simulink model "afe_abc_inv_psm_2mods"  (R2025b)
settings: Solver=ode1  StartTime=0.0  StopTime=simlength  FixedStep=tc  MaxStep=tc
values from neighbouring files (symbols this model uses):
  Adrso = eye(2) + Arso*ts_afe    [init_model.m]
  afe_pwm_phase_shift_mod1 = 0    [init_model.m]
  afe_pwm_phase_shift_mod2 = 0    [init_model.m]
  Aresd = eye(2) + Ares*ts_afe    [init_model.m]
  Bresd = Bres*ts_afe    [init_model.m]
  Cresd = Cres    [init_model.m]
  Crso = [1 0]    [init_model.m]
  CTRPIFF_CLIP_RELEASE = 0.001    [init_model.m]
  dead_time_AFE = 3e-6    (= 3e-06)    [init_model.m]
  dead_time_INV = 3e-6    (= 3e-06)    [init_model.m]
  deepNEGeta = 0.5    [init_model.m]
  deepNEGxi = 0    [init_model.m]
  deepPOSxi = 0.5    [init_model.m]
  emf_fb_p = 0.2    [init_model.m]
  emf_fb_p_ccaller_1 = emf_fb_p    (= 0.2)    [init_model.m]
  emf_fb_p_ccaller_2 = emf_fb_p    (= 0.2)    [init_model.m]
  emf_p = emf_fb_p*4/10    (= 0.08)    [init_model.m]
  emf_p_ccaller_1 = emf_fb_p_ccaller_1*4/10    (= 0.08)    [init_model.m]
  emf_p_ccaller_2 = emf_fb_p_ccaller_2*4/10    (= 0.08)    [init_model.m]
  fPWM_AFE = 4e3    (= 4000)    [init_model.m]
  fPWM_INV = fPWM_AFE    (= 4000)    [init_model.m]
  g0_161Hz = fcut_161Hz_flt * ts_afe * 2*pi    (= 0.126449104307)    [init_model.m]
  g0_1Hz = fcut_1Hz_flt * ts_afe * 2*pi    (= 0.000785398163397)    [init_model.m]
  g0_500Hz = fcut_500Hz_flt * ts_afe * 2*pi    (= 0.392699081699)    [init_model.m]
  g1_161Hz = 1 - g0_161Hz    (= 0.873550895693)    [init_model.m]
  g1_1Hz = 1 - g0_1Hz    (= 0.999214601837)    [init_model.m]
  g1_500Hz = 1 - g0_500Hz    (= 0.607300918301)    [init_model.m]
  i_grid_neg_eta_lim = 0.5    [init_model.m]
  i_grid_neg_eta_red_lim = 0.1    [init_model.m]
  i_grid_neg_xi_lim = 0.5    [init_model.m]
  i_grid_neg_xi_red_lim = 0.1    [init_model.m]
  i_grid_pos_eta_lim = 1    [init_model.m]
  i_grid_pos_eta_red_lim = 0.1    [init_model.m]
  id_lim = 0.35    [init_model.m]
  ieta_neg_ref_lim = 0.5    [init_model.m]
  ieta_pos_ref_lim = 1.0    (= 1)    [init_model.m]
  Igrid_phase_normalization_factor = 250e3/Vphase2/3/0.9*sqrt(2)    [init_model.m]
  inv_pwm_phase_shift_mod1 = 0    [init_model.m]
  iq_lim = 1.4    [init_model.m]
  ixi_pos_ref_lim = 1.6    [init_model.m]
  k_frt_ref = 2    [init_model.m]
  kg = Kobs(1)    [init_model.m]
  ki_afe = 45    [init_model.m]
  ki_align = 0.1    [init_model.m]
  ki_i = 18    [init_model.m]
  ki_rc_neg_grid = ki_rc_grid    (= 35)    [init_model.m]
  ki_rc_pos_grid = ki_rc_grid    (= 35)    [init_model.m]
  ki_vs = 35    [init_model.m]
  ki_w = 18    [init_model.m]
  kp_afe = 0.6    [init_model.m]
  kp_align = 0.6    [init_model.m]
  kp_i = 0.25    [init_model.m]
  kp_rc_neg_grid = kp_rc_grid    (= 0.35)    [init_model.m]
  kp_rc_pos_grid = kp_rc_grid    (= 0.35)    [init_model.m]
  kp_vs = 0.85    [init_model.m]
  kp_w = 2.5    [init_model.m]
  kw = Kobs(2)    [init_model.m]
  l1 = Kd(2)    [init_model.m]
  l2 = Kd(1)    [init_model.m]
  Ldrso = acker(Adrso',Crso',polesdrso)'    [init_model.m]
  lim_down_align = -0.2    [init_model.m]
  lim_up_align = 0.2    [init_model.m]
  mavarage_filter_frequency_base_order = 2    [init_model.m]
  motorc_m_scale = 2/3*Vdc_bez/ubez    [init_model.m]
  n1 = rms_perios/f_grid/ts_afe    [init_model.m]
  n10 = rms_perios/f_grid/ts_afe    [init_model.m]
  number_of_modules = 2    [init_model.m]
  omega_m_sim = omega_m_bez    [init_model.m]
  pll_i1 = 80    [init_model.m]
  pll_i1_ddsrt = pll_i1/2    (= 40)    [init_model.m]
  pll_p = 1    [init_model.m]
  pll_p_ddsrt = pll_p/2    (= 0.5)    [init_model.m]
  pll_p_frt = 0.2    [init_model.m]
  settle_time = 0.15    [init_model.m]
  simlength = 2    [init_model.m]
  start_time_LVRT = 2.0    (= 2)    [init_model.m]
  tc = ts_afe/200    (= 6.25e-07)    [init_model.m]
  time_aux_power_supply_fault = 1e3    (= 1000)    [init_model.m]
  time_gain_afe_module_1 = 1.0    (= 1)    [init_model.m]
  time_gain_afe_module_2 = 1.0    (= 1)    [init_model.m]
  time_gain_inv_module_1 = 1.0    (= 1)    [init_model.m]
  time_gain_inv_module_2 = 1.0    (= 1)    [init_model.m]
  time_phase_fault = 1e3    (= 1000)    [init_model.m]
  time_start_motor_control = 0.035    [init_model.m]
  transmission_delay = 125e-6*2    (= 0.00025)    [init_model.m]
  ts_afe = 1/fPWM_AFE/2    (= 0.000125)    [init_model.m]
  ts_inv = 1/fPWM_INV/2    (= 0.000125)    [init_model.m]
  Vdc_norm_ref = Vdc_ref/Vdc_nom    [init_model.m]
  Vdc_ref = 1070    [init_model.m]
  Vgrid_phase_normalization_factor = Vphase2*sqrt(2)    [init_model.m]
  w_grid = 2*pi*f_grid    [init_model.m]
undefined symbols (not defined in the file or in its folder): Amplitude_U, Amplitude_V, Amplitude_W, end_time_LVRT, ibez, La, Lb, Ld_norm, Lq_norm, Ls_norm, magnitude, omega_bez, omega_grid_emulator_nom, omega_grid_nom, omega_m_bez, Phase_shift, psi_bez, psi_m, psi_m_norm, rpm_base, rpm_bez, Rs, Rs_norm, t_ramp, tau_bez, torque_base, ubez, ugrid_factor, V_phase_normalization_factor, Vdc_bez, Vemu_ref_norm, vn_eta_pu, vn_xi_pu, vp_xi_pu
libraries: fl_lib x215, nesl_utility x107, simulink x22, cstblocks x20, threephase_inductor_lib x4, single_phase_transformer_lib x3, flexshaft_lib x1, psm x1
(part 9 of 19)

== system afe_abc_inv_psm_2mods/afe_abc_inv_psm_mod2/AFE_control/afe_control/FRT-VDE4110/FRT-Detection ==
  red_dyn_enabled : Inport
  Abs : Abs  SaturateOnIntegerOverflow=off
  Abs1 : Abs  SaturateOnIntegerOverflow=off
  LVRT_detector : MATLAB Function  TreatAsAtomicUnit=on
  Step1 : Step  Time=0.025  Before=1  After=0
  Step3 : Step  Time=settle_time
  dvxi_n/dt : Subsystem
  dvxi_p/dt : Subsystem
  frt_detection_inputs mod2 : Scope  NumInputPorts=6
      settings: ActiveDisplayYMinimum=-0.12991  ActiveDisplayYMaximum=1.13961  DataLoggingVariableName=ScopeData2
  frt_exceeded : Outport
  frt_state : Outport  Port=2
  red_dyn_active : Outport  Port=3
  frt_active : Outport  Port=4
  pwr_lim_enable : Outport  Port=5
  wires:
  Abs1/1 -> LVRT_detector/5(vxi_n_dot), frt_detection_inputs mod2/5  "vxi_neg_dot"
  Abs/1 -> LVRT_detector/4(vxi_p_dot), frt_detection_inputs mod2/4  "vxi_pos_dot"
  LVRT_detector/3(frt_active) -> frt_active/1
  LVRT_detector/4(frt_state) -> frt_state/1
  LVRT_detector/5(red_dyn_active) -> red_dyn_active/1
  LVRT_detector/2(frt_exceeded) -> frt_exceeded/1  "lvrt_exceeded"
  red_dyn_enabled/1 -> LVRT_detector/7(red_dyn_enabled)
  Step1/1 -> LVRT_detector/8(reset)
  dvxi_n/dt/1(xdot_hat) -> Abs1/1
  LVRT_detector/1(pwr_lim_enable) -> pwr_lim_enable/1  "pwr_lim_enable"
  dvxi_p/dt/1(xdot_hat) -> Abs/1
  Step3/1 -> LVRT_detector/6(enable), frt_detection_inputs mod2/6  "enable"
  [v_grid_neg_eta_avg_mod2] -> frt_detection_inputs mod2/3, LVRT_detector/3(veta_n)  "v_grid_neg_eta_avg"
  [v_grid_pos_xi_avg_mod2] -> dvxi_p/dt/1(x), frt_detection_inputs mod2/1, LVRT_detector/1(vxi_p)  "v_grid_pos_xi_avg"
  [v_grid_neg_xi_avg_mod2] -> dvxi_n/dt/1(x), frt_detection_inputs mod2/2, LVRT_detector/2(vxi_n)  "v_grid_neg_xi_avg"

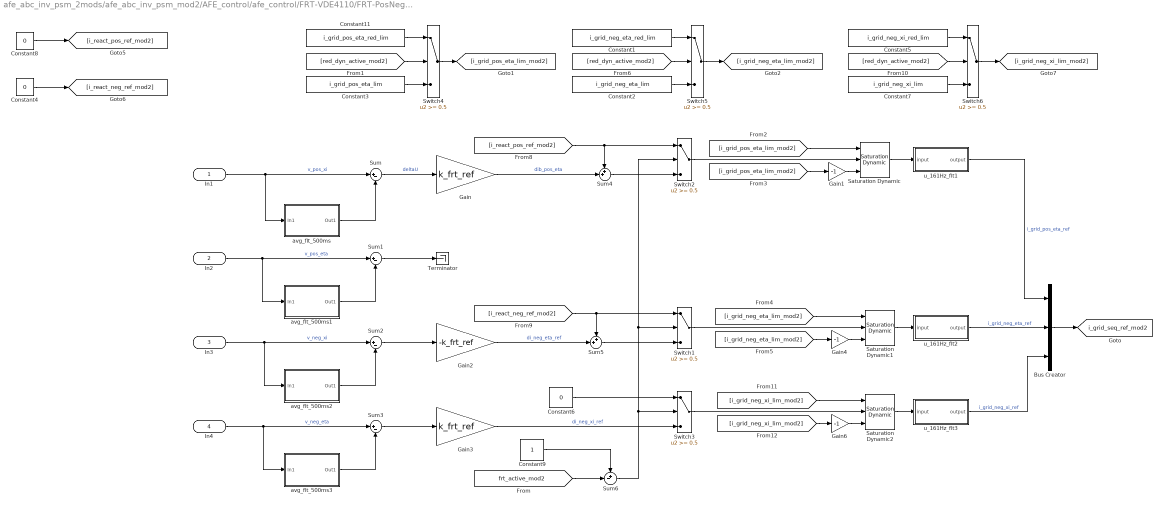
== system afe_abc_inv_psm_2mods/afe_abc_inv_psm_mod2/AFE_control/afe_control/FRT-VDE4110/FRT-PosNegReactiveCurrentReferences ==
  In1 : Inport
  In2 : Inport  Port=2
  In3 : Inport  Port=3
  In4 : Inport  Port=4
  Bus Creator : BusCreator  Inputs=3
  Constant1 : Constant  Value=i_grid_neg_eta_red_lim
  Constant11 : Constant  Value=i_grid_pos_eta_red_lim
  Constant2 : Constant  Value=i_grid_neg_eta_lim
  Constant3 : Constant  Value=i_grid_pos_eta_lim
  Constant4 : Constant  Value=0
  Constant5 : Constant  Value=i_grid_neg_xi_red_lim
  Constant6 : Constant  Value=0
  Constant7 : Constant  Value=i_grid_neg_xi_lim
  Constant8 : Constant  Value=0
  Constant9 : Constant
  Gain : Gain  Gain=k_frt_ref
  Gain1 : Gain  Gain=-1
  Gain2 : Gain  Gain=-k_frt_ref
  Gain3 : Gain  Gain=k_frt_ref
  Gain4 : Gain  Gain=-1
  Gain6 : Gain  Gain=-1
  Saturation Dynamic : simulink/Discontinuities/Saturation Dynamic  OutMin=[]  OutMax=[]  OutDataTypeStr=Inherit: Same as second input  OutDataType=fixdt(1, 16)  OutScaling=2^-10  DoSatur=off
  Saturation Dynamic1 : simulink/Discontinuities/Saturation Dynamic  OutMin=[]  OutMax=[]  OutDataTypeStr=Inherit: Same as second input  OutDataType=fixdt(1, 16)  OutScaling=2^-10  DoSatur=off
  Saturation Dynamic2 : simulink/Discontinuities/Saturation Dynamic  OutMin=[]  OutMax=[]  OutDataTypeStr=Inherit: Same as second input  OutDataType=fixdt(1, 16)  OutScaling=2^-10  DoSatur=off
  Sum{,1..3} (4 alike) : Sum  Inputs=|+-
  Sum4 : Sum  Inputs=++|
  Sum5 : Sum  Inputs=++|
  Sum6 : Sum  Inputs=+-|
  Switch{1..6} (6 alike) : Switch  Threshold=0.5  SaturateOnIntegerOverflow=off  InputSameDT=off
  Terminator : Terminator
  avg_flt_500ms : Subsystem
  avg_flt_500ms1 : Subsystem
  avg_flt_500ms2 : Subsystem
  avg_flt_500ms3 : Subsystem
  u_161Hz_flt1 : Subsystem
  u_161Hz_flt2 : Subsystem
  u_161Hz_flt3 : Subsystem
  tag scope: i_grid_seq_ref_mod2=global
  wires:
  Constant9/1 -> Sum6/1
  [frt_active_mod2] -> Sum6/2
  u_161Hz_flt1/1(output) -> Bus Creator/1  "i_grid_pos_eta_ref"
  u_161Hz_flt3/1(output) -> Bus Creator/3  "i_grid_neg_xi_ref"
  u_161Hz_flt2/1(output) -> Bus Creator/2  "i_grid_neg_eta_ref"
  Gain6/1 -> Saturation Dynamic2/3
  [red_dyn_active_mod2] -> Switch6/2
  Constant5/1 -> Switch6/1
  Switch6/1 -> [i_grid_neg_xi_lim_mod2]
  Constant7/1 -> Switch6/3
  Constant8/1 -> [i_react_pos_ref_mod2]
  Constant4/1 -> [i_react_neg_ref_mod2]
  Switch5/1 -> [i_grid_neg_eta_lim_mod2]
  Constant1/1 -> Switch5/1
  Constant2/1 -> Switch5/3
  [red_dyn_active_mod2] -> Switch5/2
  Saturation Dynamic1/1 -> u_161Hz_flt2/1(input)
  Switch1/1 -> Saturation Dynamic1/2
  [i_grid_neg_eta_lim_mod2] -> Saturation Dynamic1/1
  [i_grid_neg_eta_lim_mod2] -> Gain4/1
  Gain4/1 -> Saturation Dynamic1/3
  [i_grid_neg_xi_lim_mod2] -> Gain6/1
  [i_grid_neg_xi_lim_mod2] -> Saturation Dynamic2/1
  Switch3/1 -> Saturation Dynamic2/2
  Saturation Dynamic2/1 -> u_161Hz_flt3/1(input)
  Gain1/1 -> Saturation Dynamic/3
  [i_grid_pos_eta_lim_mod2] -> Gain1/1
  [i_grid_pos_eta_lim_mod2] -> Saturation Dynamic/1
  Constant11/1 -> Switch4/1
  Constant3/1 -> Switch4/3
  [red_dyn_active_mod2] -> Switch4/2
  Switch4/1 -> [i_grid_pos_eta_lim_mod2]
  [i_react_neg_ref_mod2] -> Sum5/1, Switch1/1
  Sum5/1 -> Switch1/3
  Gain2/1 -> Sum5/2  "di_neg_eta_ref"
  Sum3/1 -> Gain3/1
  Sum6/1 -> Switch3/2, Switch2/2, Switch1/2
  Gain3/1 -> Switch3/3  "di_neg_xi_ref"
  Constant6/1 -> Switch3/1
  Saturation Dynamic/1 -> u_161Hz_flt1/1(input)
  Switch2/1 -> Saturation Dynamic/2
  Sum4/1 -> Switch2/3
  [i_react_pos_ref_mod2] -> Sum4/1, Switch2/1
  Gain/1 -> Sum4/2  "dib_pos_eta"
  Bus Creator/1 -> [i_grid_seq_ref_mod2]
  In4/1 -> Sum3/1, avg_flt_500ms3/1(In1)  "v_neg_eta"
  avg_flt_500ms2/1(Out1) -> Sum2/2
  In3/1 -> Sum2/1, avg_flt_500ms2/1(In1)  "v_neg_xi"
  Sum2/1 -> Gain2/1
  avg_flt_500ms3/1(Out1) -> Sum3/2
  In2/1 -> Sum1/1, avg_flt_500ms1/1(In1)  "v_pos_eta"
  avg_flt_500ms1/1(Out1) -> Sum1/2
  Sum1/1 -> Terminator/1
  Sum/1 -> Gain/1  "deltaU"
  avg_flt_500ms/1(Out1) -> Sum/2
  In1/1 -> Sum/1, avg_flt_500ms/1(In1)  "v_pos_xi"

== system afe_abc_inv_psm_2mods/afe_abc_inv_psm_mod2/AFE_control/afe_control/current_ctrl/Inner Loop Current Control ==
  In1 : Inport
  is_abc : Inport  Port=2
  -1<x<1 : Saturate  UpperLimit=1  LowerLimit=-1
  Add : Sum
  Bus Creator1 : BusCreator  Inputs=2
  "Current-Control, Phase a" : Subsystem
  "Current-Control, Phase b" : Subsystem
  "Current-Control, Phase c" : Subsystem
  Demux1 : Demux  Outputs=3
  MATLAB Function : MATLAB Function  TreatAsAtomicUnit=on
  Mux : Mux  Inputs=3
  Selector : Selector  InputPortWidth=3  IndexOptions=Index vector (dialog)  Indices=[1]  OutputSizes=1
  Selector1 : Selector  InputPortWidth=3  IndexOptions=Index vector (dialog)  Indices=[1]  OutputSizes=1
  Selector2 : Selector  InputPortWidth=3  IndexOptions=Index vector (dialog)  Indices=[2]  OutputSizes=1
  Selector3 : Selector  InputPortWidth=3  IndexOptions=Index vector (dialog)  Indices=[2]  OutputSizes=1
  Selector4 : Selector  InputPortWidth=3  IndexOptions=Index vector (dialog)  Indices=[3]  OutputSizes=1
  Selector5 : Selector  InputPortWidth=3  IndexOptions=Index vector (dialog)  Indices=[3]  OutputSizes=1
  To Workspace1 : ToWorkspace  VariableName=isa_ref_sim_mod2  SampleTime=-1
      settings: MaxDataPoints=Ns_afe
  To Workspace2 : ToWorkspace  VariableName=isa_sim_mod2  SampleTime=-1
      settings: MaxDataPoints=Ns_afe
  To Workspace3 : ToWorkspace  VariableName=isb_ref_sim_mod2  SampleTime=-1
      settings: MaxDataPoints=Ns_afe
  To Workspace4 : ToWorkspace  VariableName=isb_sim_mod2  SampleTime=-1
      settings: MaxDataPoints=Ns_afe
  To Workspace5 : ToWorkspace  VariableName=isc_ref_sim_mod2  SampleTime=-1
      settings: MaxDataPoints=Ns_afe
  To Workspace6 : ToWorkspace  VariableName=isc_sim_mod2  SampleTime=-1
      settings: MaxDataPoints=Ns_afe
  Unit Delay1 : UnitDelay  SampleTime=-1  HasFrameUpgradeWarning=on
  Unit Delay2 : UnitDelay  SampleTime=-1  HasFrameUpgradeWarning=on
  Unit Delay3 : UnitDelay  SampleTime=-1  HasFrameUpgradeWarning=on
  afe_ictrl_out/afe_ictrl_ff : Scope  NumInputPorts=2
      settings: ActiveDisplayYMinimum=-1.2844276731305864  ActiveDisplayYMaximum=1.2966894715372321  DataLoggingVariableName=ScopeData4
  isa_ref/isa : Scope  NumInputPorts=2
      settings: ActiveDisplayYMinimum=-1.06078125  ActiveDisplayYMaximum=1.00328125
  isb_ref/isb : Scope  NumInputPorts=2
      settings: ActiveDisplayYMinimum=-1.080322265625  ActiveDisplayYMaximum=1.007080078125  DataLoggingVariableName=ScopeData2
  isc_ref/isc : Scope  NumInputPorts=2
      settings: ActiveDisplayYMinimum=-1.005859375  ActiveDisplayYMaximum=1.0791015625  DataLoggingVariableName=ScopeData3
  uab : Outport  VectorParamsAs1DForOutWhenUnconnected=off
  wires:
  [isc_mod2] -> To Workspace6/1
  [isc_ref_mod2] -> To Workspace5/1
  [isb_ref_mod2] -> To Workspace3/1
  [isb_mod2] -> To Workspace4/1
  [isa_mod2] -> To Workspace2/1
  [isa_ref_mod2] -> To Workspace1/1
  [v_grid_ff_abc_mod2] -> Unit Delay1/1
  Unit Delay1/1 -> afe_ictrl_out/afe_ictrl_ff/2  "v_grid_ff_abc_mod1"
  -1<x<1/1 -> Demux1/1  "v_abc"
  Bus Creator1/1 -> uab/1
  Unit Delay2/1 -> Bus Creator1/1  "ualpha_afe"
  Demux1/1 -> MATLAB Function/1(a)  "v_a"
  MATLAB Function/2(beta) -> Unit Delay3/1  "u_beta"
  Demux1/2 -> MATLAB Function/2(b)  "v_b"
  Unit Delay3/1 -> Bus Creator1/2  "ubeta_afe"
  MATLAB Function/1(alpha) -> Unit Delay2/1  "u_alpha"
  Demux1/3 -> MATLAB Function/3(c)  "v_c"
  Mux/1 -> afe_ictrl_out/afe_ictrl_ff/1, Add/1  "v_abc"
  "Current-Control, Phase c"/1(Out1) -> Mux/3  "v_c"
  "Current-Control, Phase b"/1(Out1) -> Mux/2  "v_b"
  "Current-Control, Phase a"/1(Out1) -> Mux/1  "v_a"
  Selector5/1 -> "Current-Control, Phase c"/2(In2), [isc_mod2], isc_ref/isc/2  "isc"
  Selector4/1 -> "Current-Control, Phase c"/1(In1), [isc_ref_mod2], isc_ref/isc/1  "isc_ref"
  Selector3/1 -> "Current-Control, Phase b"/2(In2), isb_ref/isb/2, [isb_mod2]  "isb"
  Selector2/1 -> "Current-Control, Phase b"/1(In1), isb_ref/isb/1, [isb_ref_mod2]  "isb_ref"
  Selector1/1 -> "Current-Control, Phase a"/2(In2), isa_ref/isa/2, [isa_mod2]  "isa"
  Selector/1 -> "Current-Control, Phase a"/1(In1), [isa_ref_mod2], isa_ref/isa/1  "isa_ref"
  Add/1 -> -1<x<1/1  "v_abc"
  is_abc/1 -> Selector1/1, Selector3/1, Selector5/1  "id_abc"
  In1/1 -> Selector/1, Selector2/1, Selector4/1  "id_abc_ref"

== system afe_abc_inv_psm_2mods/afe_abc_inv_psm_mod2/AFE_control/afe_control/current_ctrl/current_transformation ==
  is_a_pu : Inport
  is_b_pu : Inport  Port=2
  is_c_pu : Inport  Port=3
  alphabeta2xieta : MATLAB Function  TreatAsAtomicUnit=on
  uvw2alphabeta : MATLAB Function  TreatAsAtomicUnit=on
  tag scope: id_eta_pu_mod2=global, id_xi_pu_mod2=global
  wires:
  is_a_pu/1 -> uvw2alphabeta/1(u)
  [gamma_grid_pll_mod2] -> alphabeta2xieta/3(gamma)
  uvw2alphabeta/1(alpha) -> alphabeta2xieta/1(alpha)  "ialpha_pu"
  uvw2alphabeta/2(beta) -> alphabeta2xieta/2(beta)  "ibeta_pu"
  is_b_pu/1 -> uvw2alphabeta/2(v)
  alphabeta2xieta/1(xi) -> [id_xi_pu_mod2]  "ixi_pu"
  alphabeta2xieta/2(eta) -> [id_eta_pu_mod2]  "ieta_pu"
  is_c_pu/1 -> uvw2alphabeta/3(w)

== system afe_abc_inv_psm_2mods/afe_abc_inv_psm_mod2/AFE_control/afe_control/current_ctrl/xieta2abc ==
  pos_xi : Inport
  pos_eta : Inport  Port=2
  neg_xi : Inport  Port=3
  neg_eta : Inport  Port=4
  gamma : Inport  Port=5
  MATLAB Function2 : MATLAB Function  TreatAsAtomicUnit=on
  Mux : Mux  Inputs=3
  Negative Sequence : MATLAB Function  TreatAsAtomicUnit=on
  Positive Sequence : MATLAB Function  TreatAsAtomicUnit=on
  Sum : Sum  Inputs=|++
  Sum1 : Sum  Inputs=|++
  i_abc : Outport
  wires:
  Mux/1 -> i_abc/1  "i_abc"
  pos_eta/1 -> Positive Sequence/2(eta)
  pos_xi/1 -> Positive Sequence/1(xi)
  neg_xi/1 -> Negative Sequence/1(xi)
  Sum1/1 -> MATLAB Function2/2(beta)
  MATLAB Function2/2(b) -> Mux/2  "i_b"
  Negative Sequence/2(beta) -> Sum1/2
  Positive Sequence/1(alpha) -> Sum/1
  Negative Sequence/1(alpha) -> Sum/2
  MATLAB Function2/3(c) -> Mux/3  "i_c"
  gamma/1 -> Positive Sequence/3(gamma), Negative Sequence/3(gamma)
  Sum/1 -> MATLAB Function2/1(alpha)
  Positive Sequence/2(beta) -> Sum1/1
  MATLAB Function2/1(a) -> Mux/1  "i_a"
  neg_eta/1 -> Negative Sequence/2(eta)

== system afe_abc_inv_psm_2mods/afe_abc_inv_psm_mod2/AFE_control/afe_control/grid_current_sequences_and_reactive_pwr_ctrl/current_sequence_avg ==
  i_grid_pos_xi : Inport
  i_grid_pos_eta : Inport  Port=2
  i_grid_neg_xi : Inport  Port=3
  i_grid_neg_eta : Inport  Port=4
  Variant Source{,1..3} (4 alike) : VariantSource  VariantControls={use_moving_average_from_ccaller_mod2 == 1, use_moving_average_from_ccaller_mod2 == 0}
  average_filter_ccaller : Subsystem  Commented=on
  average_filter_simulink : Subsystem
  i_grid_pos_xi_avg : Outport
  i_grid_pos_eta_avg : Outport  Port=2
  i_grid_neg_xi_avg : Outport  Port=3
  i_grid_neg_eta_avg : Outport  Port=4
  wires:
  average_filter_ccaller/4(i_grid_neg_eta_avg) -> Variant Source3/1
  average_filter_ccaller/3(i_grid_neg_xi_avg) -> Variant Source2/1
  average_filter_ccaller/2(i_grid_pos_eta_avg) -> Variant Source1/1
  average_filter_simulink/4(i_grid_neg_eta_avg) -> Variant Source3/2
  average_filter_simulink/3(i_grid_neg_xi_avg) -> Variant Source2/2
  average_filter_simulink/2(i_grid_pos_eta_avg) -> Variant Source1/2
  average_filter_simulink/1(i_grid_pos_xi_avg) -> Variant Source/2
  average_filter_ccaller/1(i_grid_pos_xi_avg) -> Variant Source/1
  Variant Source1/1 -> i_grid_pos_eta_avg/1
  Variant Source2/1 -> i_grid_neg_xi_avg/1
  Variant Source3/1 -> i_grid_neg_eta_avg/1
  Variant Source/1 -> i_grid_pos_xi_avg/1
  i_grid_neg_eta/1 -> average_filter_ccaller/4(i_grid_neg_eta), average_filter_simulink/4(i_grid_neg_eta)
  i_grid_neg_xi/1 -> average_filter_ccaller/3(i_grid_neg_xi), average_filter_simulink/3(i_grid_neg_xi)
  i_grid_pos_eta/1 -> average_filter_ccaller/2(i_grid_pos_eta), average_filter_simulink/2(i_grid_pos_eta)
  i_grid_pos_xi/1 -> average_filter_ccaller/1(i_grid_pos_xi), average_filter_simulink/1(i_grid_pos_xi)

== system afe_abc_inv_psm_2mods/afe_abc_inv_psm_mod2/AFE_control/afe_control/grid_current_sequences_and_reactive_pwr_ctrl/grid_current_sampling_and_alpha_beta_transformation ==
  ig_abc : Inport
  i_abc2alphabeta : MATLAB Function  TreatAsAtomicUnit=on
  i_grid_alpha : Outport
  i_grid_beta : Outport  Port=2
  wires:
  ig_abc/1 -> i_abc2alphabeta/1(i_abc)
  i_abc2alphabeta/1(alpha) -> i_grid_alpha/1  "i_grid_alpha"
  i_abc2alphabeta/2(beta) -> i_grid_beta/1  "i_grid_beta"

== system afe_abc_inv_psm_2mods/afe_abc_inv_psm_mod2/AFE_control/afe_control/grid_current_sequences_and_reactive_pwr_ctrl/i_alphabeta2xieta ==
  alpha : Inport
  beta : Inport  Port=2
  gamma : Inport  Port=3
  MATLAB Function : MATLAB Function  TreatAsAtomicUnit=on
  MATLAB Function1 : MATLAB Function  TreatAsAtomicUnit=on
  xi : Outport
  v_grid_pos_eta : Outport  Port=2
  v_grid_neg_xi : Outport  Port=3
  e : Outport  Port=4
  wires:
  MATLAB Function/1(xi) -> xi/1  "i_grid_pos_xi"
  MATLAB Function1/2(eta) -> e/1  "i_grid_neg_eta"
  MATLAB Function1/1(xi) -> v_grid_neg_xi/1  "i_grid_neg_xi"
  MATLAB Function/2(eta) -> v_grid_pos_eta/1  "i_grid_pos_eta"
  gamma/1 -> MATLAB Function/3(gamma), MATLAB Function1/3(gamma)  "gamma_grid"
  beta/1 -> MATLAB Function/2(beta), MATLAB Function1/2(beta)  "i_grid_beta"
  alpha/1 -> MATLAB Function/1(alpha), MATLAB Function1/1(alpha)  "i_grid_alpha"

== system afe_abc_inv_psm_2mods/afe_abc_inv_psm_mod2/AFE_control/afe_control/grid_current_sequences_and_reactive_pwr_ctrl/sequences_current_control ==
  i_pos_xi : Inport
  i_pos_eta : Inport  Port=2
  i_neg_xi : Inport  Port=3
  i_neg_eta : Inport  Port=4
  Bus Selector : BusSelector  OutputSignals=i_grid_pos_eta_ref,i_grid_neg_eta_ref,i_grid_neg_xi_ref
  Gain : Gain  Gain=-1
  Gain1 : Gain  Gain=-1
  Gain2 : Gain  Gain=-1
  Negative-Seq. eta-Control : Subsystem
  Negative-Seq. xi-Control : Subsystem
  Positive-Seq. eta-Control : Subsystem
  Sum : Sum  Inputs=|+-
  Sum1 : Sum  Inputs=|+-
  Sum2 : Sum  Inputs=|+-
  Terminator : Terminator
  i_neg_eta_ref/i_neg_eta mod2 : Scope  NumInputPorts=2
      settings: ActiveDisplayYMinimum=-1  ActiveDisplayYMaximum=1  DataLoggingVariableName=ScopeData6
  i_neg_xi_ref/i_neg_xi mod2 : Scope  NumInputPorts=2
      settings: ActiveDisplayYMinimum=-0.093272384387596066  ActiveDisplayYMaximum=0.21232485707584112  DataLoggingVariableName=ScopeData7
  i_pos_eta_ref/i_pos_eta mod2 : Scope  NumInputPorts=2
      settings: ActiveDisplayYMinimum=-0.13263870980821479  ActiveDisplayYMaximum=0.34001616382199712  DataLoggingVariableName=ScopeData5
  tag scope: i_stack_neg_eta_ref_mod2=global, i_stack_neg_xi_ref_mod2=global, i_stack_pos_eta_ref_mod2=global
  wires:
  Negative-Seq. xi-Control/1(u) -> [i_stack_neg_xi_ref_mod2]
  Negative-Seq. eta-Control/1(u) -> [i_stack_neg_eta_ref_mod2]
  Positive-Seq. eta-Control/1(u) -> [i_stack_pos_eta_ref_mod2]
  Gain2/1 -> Negative-Seq. xi-Control/2(e)
  Gain1/1 -> Negative-Seq. eta-Control/2(e)
  Gain/1 -> Positive-Seq. eta-Control/2(e)
  i_neg_xi/1 -> Sum2/2, i_neg_xi_ref/i_neg_xi mod2/2  "i_neg_xi"
  i_neg_eta/1 -> i_neg_eta_ref/i_neg_eta mod2/2, Sum1/2  "i_neg_eta"
  i_pos_eta/1 -> Sum/2, i_pos_eta_ref/i_pos_eta mod2/2  "i_pos_eta"
  Sum/1 -> Gain/1
  Sum1/1 -> Gain1/1
  Sum2/1 -> Gain2/1
  Bus Selector/3 -> Sum2/1, i_neg_xi_ref/i_neg_xi mod2/1  "<i_grid_neg_xi_ref>"
  Bus Selector/2 -> i_neg_eta_ref/i_neg_eta mod2/1, Sum1/1  "<i_grid_neg_eta_ref>"
  Bus Selector/1 -> Sum/1, i_pos_eta_ref/i_pos_eta mod2/1  "<i_grid_pos_eta_ref>"
  [i_grid_seq_ref_mod2] -> Bus Selector/1
  i_pos_xi/1 -> Terminator/1

== system afe_abc_inv_psm_2mods/afe_abc_inv_psm_mod2/AFE_control/afe_control/grid_voltage_phase_lock_loops/DDSRF-PLL ==
  ug_abc_pu : Inport
  pll_stageA : Subsystem
  pll_stageB : Subsystem
  gamma_grid_ddsrf_pll : Outport
  omega_grid_ddsrf_pll : Outport  Port=2
  wires:
  ug_abc_pu/1 -> pll_stageA/2(ug_abc_pu)
  pll_stageB/2(omega_grid_ddsrf_pll) -> omega_grid_ddsrf_pll/1
  pll_stageA/1(u_grid_pos_xi) -> pll_stageB/1(u_grid_pos_xi)  "u_grid_pos_xi"
  pll_stageA/2(u_grid_pos_eta) -> pll_stageB/2(u_grid_pos_eta)  "u_grid_pos_eta"
  pll_stageB/1(gamma_grid_ddsrf_pll) -> gamma_grid_ddsrf_pll/1, pll_stageA/1(gamma_grid)

== system afe_abc_inv_psm_2mods/afe_abc_inv_psm_mod2/AFE_control/afe_control/grid_voltage_phase_lock_loops/dq_pll ==
  ug_abc_pu : Inport
  pll_stageA : Subsystem
  pll_stageB : Subsystem
  gamma_grid_dqpll : Outport
  omega_grid_dqpll : Outport  Port=2
  wires:
  ug_abc_pu/1 -> pll_stageA/2(ug_abc)
  pll_stageB/2(omega_grid_pll) -> omega_grid_dqpll/1
  pll_stageA/1(u_grid_pos_xi) -> pll_stageB/1(u_grid_pos_xi)  "u_grid_pos_xi"
  pll_stageB/1(gamma_grid_pll) -> pll_stageA/1(gamma_grid), gamma_grid_dqpll/1
  pll_stageA/2(u_grid_pos_eta) -> pll_stageB/2(u_grid_pos_eta)  "u_grid_pos_eta"

== system afe_abc_inv_psm_2mods/afe_abc_inv_psm_mod2/AFE_control/afe_control/grid_voltage_phase_lock_loops/dq_pll_ccaller ==
  ug_abc_pu : Inport
  Bus Selector : BusSelector  OutputSignals=omega_pu_hat,gamma_hat,u_grid_xi,u_grid_eta,dqpll_pll_state
  C Caller : CCaller  FunctionName=dqpll_grid_process_simulink  PortSpecificationStruct="%)30     .    N H   8    (     @         %    \"     8    !     0         %  0 \"0    $    _    07)G3F%M90  4&]R=$YA;64 4V-O<&4     26YD97@     5'EP90      4VEZ90      27-';&]B86P   X    P    !@    @    $          4    (     0    ,    !         !   P!O=70 #@   #     &    \"     0         !0    @    !     P    $         $  # &]U=  .    .     8    (    !          %    \"     $    &     0         0   ...(+3319 chars)"
  Constant : Constant  Value=ts_afe
  Data Type Conversion{1..2,4..5} (4 alike) : DataTypeConversion  OutDataTypeStr=single  SaturateOnIntegerOverflow=off  RndMeth=Floor
  Data Type Conversion{6..10} (5 alike) : DataTypeConversion  OutDataTypeStr=double  SaturateOnIntegerOverflow=off  RndMeth=Floor
  Data Type Conversion3 : DataTypeConversion  OutDataTypeStr=uint8  SaturateOnIntegerOverflow=off  RndMeth=Floor
  Demux : Demux  Outputs=3
  Step : Step  Time=0.01  Before=1  After=0
  first_harmonic_tracker mod2 : Scope  NumInputPorts=3
      settings: ActiveDisplayYMinimum=-1.7184470891952515  ActiveDisplayYMaximum=1.8384636640548706
  first_harmonic_tracker_phase_u : Subsystem
  first_harmonic_tracker_phase_v : Subsystem
  first_harmonic_tracker_phase_w : Subsystem
  gamma_hat : Outport  VectorParamsAs1DForOutWhenUnconnected=off
  omega_pu_hat : Outport  Port=2  VectorParamsAs1DForOutWhenUnconnected=off
  dqpll_uxi : Outport  Port=3  VectorParamsAs1DForOutWhenUnconnected=off
  dqpll_ueta : Outport  Port=4  VectorParamsAs1DForOutWhenUnconnected=off
  dqpll_state : Outport  Port=5  VectorParamsAs1DForOutWhenUnconnected=off
  wires:
  first_harmonic_tracker_phase_w/1(u_hat) -> Data Type Conversion5/1, first_harmonic_tracker mod2/3  "tracker_phase_w"
  first_harmonic_tracker_phase_v/1(u_hat) -> Data Type Conversion4/1, first_harmonic_tracker mod2/2  "tracker_phase_v"
  first_harmonic_tracker_phase_u/1(u_hat) -> Data Type Conversion2/1, first_harmonic_tracker mod2/1  "tracker_phase_u"
  Data Type Conversion6/1 -> omega_pu_hat/1
  Demux/3 -> first_harmonic_tracker_phase_w/1(u)
  Demux/2 -> first_harmonic_tracker_phase_v/1(u)
  Demux/1 -> first_harmonic_tracker_phase_u/1(u)
  ug_abc_pu/1 -> Demux/1
  Data Type Conversion9/1 -> dqpll_ueta/1
  Data Type Conversion8/1 -> dqpll_uxi/1
  Data Type Conversion10/1 -> dqpll_state/1
  Data Type Conversion7/1 -> gamma_hat/1
  Bus Selector/5 -> Data Type Conversion10/1  "<dqpll_pll_state>"
  Bus Selector/4 -> Data Type Conversion9/1  "<u_grid_eta>"
  Bus Selector/3 -> Data Type Conversion8/1  "<u_grid_xi>"
  Bus Selector/2 -> Data Type Conversion7/1  "<gamma_hat>"
  Bus Selector/1 -> Data Type Conversion6/1  "<omega_pu_hat>"
  C Caller/1 -> Bus Selector/1
  Data Type Conversion1/1 -> C Caller/5
  Data Type Conversion5/1 -> C Caller/4
  Data Type Conversion4/1 -> C Caller/3
  Data Type Conversion2/1 -> C Caller/2
  Data Type Conversion3/1 -> C Caller/1
  Constant/1 -> Data Type Conversion1/1
  Step/1 -> Data Type Conversion3/1

== system afe_abc_inv_psm_2mods/afe_abc_inv_psm_mod2/AFE_control/afe_control/grid_voltage_sequences/grid_voltage_sampling_and_alpha_beta_transformation ==
  v_abc : Inport
  v_abc2alphabeta : MATLAB Function  TreatAsAtomicUnit=on
  u_grid_alpha : Outport
  u_grid_beta : Outport  Port=2
  wires:
  v_abc/1 -> v_abc2alphabeta/1(v_abc)
  v_abc2alphabeta/2(beta) -> u_grid_beta/1  "u_grid_beta"
  v_abc2alphabeta/1(alpha) -> u_grid_alpha/1  "u_grid_alpha"

== system afe_abc_inv_psm_2mods/afe_abc_inv_psm_mod2/AFE_control/afe_control/grid_voltage_sequences/v_alphabeta2xieta ==
  alpha : Inport
  beta : Inport  Port=2
  gamma : Inport  Port=3
  MATLAB Function : MATLAB Function  TreatAsAtomicUnit=on
  MATLAB Function1 : MATLAB Function  TreatAsAtomicUnit=on
  xi : Outport
  eta : Outport  Port=2
  v_grid_neg_xi : Outport  Port=3
  v_grid_neg_eta : Outport  Port=4
  wires:
  MATLAB Function1/2(eta) -> v_grid_neg_eta/1  "u_grid_neg_eta"
  MATLAB Function1/1(xi) -> v_grid_neg_xi/1  "u_grid_neg_xi"
  MATLAB Function/2(eta) -> eta/1  "u_grid_pos_eta"
  MATLAB Function/1(xi) -> xi/1  "u_grid_pos_xi"
  gamma/1 -> MATLAB Function/3(gamma), MATLAB Function1/3(gamma)  "gamma_grid"
  beta/1 -> MATLAB Function/2(beta), MATLAB Function1/2(beta)  "u_grid_beta"
  alpha/1 -> MATLAB Function/1(alpha), MATLAB Function1/1(alpha)  "u_grid_alpha"

== system afe_abc_inv_psm_2mods/afe_abc_inv_psm_mod2/AFE_control/afe_control/grid_voltage_sequences/voltage_sequence_avg ==
  v_grid_pos_xi : Inport
  v_grid_pos_eta : Inport  Port=2
  v_grid_neg_xi : Inport  Port=3
  v_grid_neg_eta : Inport  Port=4
  Variant Source{1..4} (4 alike) : VariantSource  VariantControls={use_moving_average_from_ccaller_mod2 == 1, use_moving_average_from_ccaller_mod2 == 0}
  average_filter_ccaller : Subsystem  Commented=on
  average_filter_simulink : Subsystem
  v_grid_pos_xi_avg : Outport
  v_grid_pos_eta_avg : Outport  Port=2
  v_grid_neg_xi_avg : Outport  Port=3
  v_grid_neg_eta_avg : Outport  Port=4
  wires:
  average_filter_simulink/4(v_grid_neg_eta_avg) -> Variant Source3/2
  average_filter_simulink/3(v_grid_neg_xi_avg) -> Variant Source2/2
  average_filter_simulink/2(v_grid_pos_eta_avg) -> Variant Source1/2
  average_filter_simulink/1(v_grid_pos_xi_avg) -> Variant Source4/2
  average_filter_ccaller/4(v_grid_neg_eta_avg) -> Variant Source3/1
  average_filter_ccaller/3(v_grid_neg_xi_avg) -> Variant Source2/1
  average_filter_ccaller/2(v_grid_pos_eta_avg) -> Variant Source1/1
  average_filter_ccaller/1(v_grid_pos_xi_avg) -> Variant Source4/1
  Variant Source3/1 -> v_grid_neg_eta_avg/1
  Variant Source2/1 -> v_grid_neg_xi_avg/1
  Variant Source1/1 -> v_grid_pos_eta_avg/1
  Variant Source4/1 -> v_grid_pos_xi_avg/1
  v_grid_neg_eta/1 -> average_filter_ccaller/4(v_grid_neg_eta), average_filter_simulink/4(v_grid_neg_eta)
  v_grid_neg_xi/1 -> average_filter_ccaller/3(v_grid_neg_xi), average_filter_simulink/3(v_grid_neg_xi)
  v_grid_pos_eta/1 -> average_filter_ccaller/2(v_grid_pos_eta), average_filter_simulink/2(v_grid_pos_eta)
  v_grid_pos_xi/1 -> average_filter_ccaller/1(v_grid_pos_xi), average_filter_simulink/1(v_grid_pos_xi)

== system afe_abc_inv_psm_2mods/afe_abc_inv_psm_mod2/AFE_control/afe_control/ig afe quantizzation and one step delay/ig afe quantizzation and one step delay ==
  ig_u_pu : Inport
  ig_v_pu : Inport  Port=2
  ig_w_pu : Inport  Port=3
  Gain4 : Gain  Gain=-1
  Gain5 : Gain  Gain=-1
  Gain6 : Gain  Gain=-1
  Quantizer1 : Quantizer  QuantizationInterval=adc_quantization
  Quantizer2 : Quantizer  QuantizationInterval=adc_quantization
  Quantizer4 : Quantizer  QuantizationInterval=adc_quantization
  Unit Delay : UnitDelay  SampleTime=-1  HasFrameUpgradeWarning=on
  Unit Delay1 : UnitDelay  SampleTime=-1  HasFrameUpgradeWarning=on
  Unit Delay2 : UnitDelay  SampleTime=-1  HasFrameUpgradeWarning=on
  igd_u_pu : Outport
  igd_v_pu : Outport  Port=2
  igd_w_pu : Outport  Port=3
  wires:
  Gain6/1 -> igd_w_pu/1
  Gain5/1 -> igd_v_pu/1
  Gain4/1 -> igd_u_pu/1
  Unit Delay2/1 -> Gain6/1
  Unit Delay1/1 -> Gain5/1
  Unit Delay/1 -> Gain4/1
  ig_w_pu/1 -> Quantizer2/1
  ig_v_pu/1 -> Quantizer1/1
  ig_u_pu/1 -> Quantizer4/1
  Quantizer2/1 -> Unit Delay2/1
  Quantizer4/1 -> Unit Delay/1
  Quantizer1/1 -> Unit Delay1/1

== system afe_abc_inv_psm_2mods/afe_abc_inv_psm_mod2/AFE_control/afe_control/instantaneus_power/abc2alphabeta ==
  a : Inport
  b : Inport  Port=2
  c : Inport  Port=3
  Gain1 : Gain  Gain=-1/2
  Gain11 : Gain  Gain=-1/2
  Gain2 : Gain  Gain=0
  Gain3 : Gain  Gain=sqrt(3)/2
  Gain4 : Gain  Gain=-sqrt(3)/2
  Gain8 : Gain  Gain=2/3
  Gain9 : Gain  Gain=2/3
  Sum : Sum  Inputs=+++
  Sum1 : Sum  Inputs=+++
  "alpha " : Outport  VectorParamsAs1DForOutWhenUnconnected=off
  "beta " : Outport  Port=2  VectorParamsAs1DForOutWhenUnconnected=off
  wires:
  a/1 -> Sum/1, Gain2/1
  Gain1/1 -> Sum/3
  b/1 -> Gain11/1, Gain3/1
  Gain9/1 -> "beta "/1
  c/1 -> Gain1/1, Gain4/1
  Sum/1 -> Gain8/1
  Gain8/1 -> "alpha "/1
  Sum1/1 -> Gain9/1
  Gain4/1 -> Sum1/3
  Gain11/1 -> Sum/2
  Gain2/1 -> Sum1/1
  Gain3/1 -> Sum1/2

== system afe_abc_inv_psm_2mods/afe_abc_inv_psm_mod2/AFE_control/afe_control/instantaneus_power/abc2alphabeta  ==
  a : Inport
  b : Inport  Port=2
  c : Inport  Port=3
  Gain1 : Gain  Gain=-1/2
  Gain11 : Gain  Gain=-1/2
  Gain2 : Gain  Gain=0
  Gain3 : Gain  Gain=sqrt(3)/2
  Gain4 : Gain  Gain=-sqrt(3)/2
  Gain8 : Gain  Gain=2/3
  Gain9 : Gain  Gain=2/3
  Sum : Sum  Inputs=+++
  Sum1 : Sum  Inputs=+++
  "alpha " : Outport  VectorParamsAs1DForOutWhenUnconnected=off
  "beta " : Outport  Port=2  VectorParamsAs1DForOutWhenUnconnected=off
  wires:
  b/1 -> Gain3/1, Gain11/1
  Gain8/1 -> "alpha "/1
  Gain4/1 -> Sum1/3
  Gain3/1 -> Sum1/2
  Gain1/1 -> Sum/3
  Sum1/1 -> Gain9/1
  Sum/1 -> Gain8/1
  c/1 -> Gain4/1, Gain1/1
  Gain11/1 -> Sum/2
  Gain9/1 -> "beta "/1
  Gain2/1 -> Sum1/1
  a/1 -> Gain2/1, Sum/1

== system afe_abc_inv_psm_2mods/afe_abc_inv_psm_mod2/AFE_control/afe_control/instantaneus_power/moving_avarage_p ==
  in : Inport
  Gain : Gain  Gain=n1-1
  Gain1 : Gain  Gain=1/n1
  Sum : Sum  Inputs=|++
  Unit Delay : UnitDelay  SampleTime=-1  HasFrameUpgradeWarning=on
  out : Outport  VectorParamsAs1DForOutWhenUnconnected=off
  wires:
  Sum/1 -> Gain1/1
  Unit Delay/1 -> Gain/1
  in/1 -> Sum/1
  Gain1/1 -> Unit Delay/1, out/1
  Gain/1 -> Sum/2

== system afe_abc_inv_psm_2mods/afe_abc_inv_psm_mod2/AFE_control/afe_control/instantaneus_power/moving_avarage_q ==
  in : Inport
  Gain : Gain  Gain=n1-1
  Gain1 : Gain  Gain=1/n1
  Sum : Sum  Inputs=|++
  Unit Delay : UnitDelay  SampleTime=-1  HasFrameUpgradeWarning=on
  out : Outport  VectorParamsAs1DForOutWhenUnconnected=off
  wires:
  Gain/1 -> Sum/2
  Gain1/1 -> out/1, Unit Delay/1
  in/1 -> Sum/1
  Unit Delay/1 -> Gain/1
  Sum/1 -> Gain1/1

== system afe_abc_inv_psm_2mods/afe_abc_inv_psm_mod2/AFE_control/afe_control/instantaneus_power/rms ==
  In1 : Inport
  Gain : Gain  Gain=n10-1
  Gain1 : Gain  Gain=1/n10
  Math Function : Math  Operator=magnitude^2  SignedPower=on
  Sqrt : Sqrt
  Sum : Sum  Inputs=|++
  Unit Delay : UnitDelay  SampleTime=-1  HasFrameUpgradeWarning=on
  Out1 : Outport  VectorParamsAs1DForOutWhenUnconnected=off
  wires:
  Gain/1 -> Sum/2
  Sqrt/1 -> Out1/1
  Math Function/1 -> Sum/1
  Unit Delay/1 -> Gain/1
  Gain1/1 -> Unit Delay/1, Sqrt/1
  Sum/1 -> Gain1/1
  In1/1 -> Math Function/1

== system afe_abc_inv_psm_2mods/afe_abc_inv_psm_mod2/AFE_control/afe_control/instantaneus_power/rms1 ==
  In1 : Inport
  Gain : Gain  Gain=n10-1
  Gain1 : Gain  Gain=1/n10
  Math Function : Math  Operator=magnitude^2  SignedPower=on
  Sqrt : Sqrt
  Sum : Sum  Inputs=|++
  Unit Delay : UnitDelay  SampleTime=-1  HasFrameUpgradeWarning=on
  Out1 : Outport  VectorParamsAs1DForOutWhenUnconnected=off
  wires:
  In1/1 -> Math Function/1
  Sum/1 -> Gain1/1
  Gain1/1 -> Sqrt/1, Unit Delay/1
  Unit Delay/1 -> Gain/1
  Math Function/1 -> Sum/1
  Sqrt/1 -> Out1/1
  Gain/1 -> Sum/2

== system afe_abc_inv_psm_2mods/afe_abc_inv_psm_mod2/AFE_control/afe_control/instantaneus_power/rms2 ==
  In1 : Inport
  Gain : Gain  Gain=n10-1
  Gain1 : Gain  Gain=1/n10
  Math Function : Math  Operator=magnitude^2  SignedPower=on
  Sqrt : Sqrt
  Sum : Sum  Inputs=|++
  Unit Delay : UnitDelay  SampleTime=-1  HasFrameUpgradeWarning=on
  Out1 : Outport  VectorParamsAs1DForOutWhenUnconnected=off
  wires:
  Gain/1 -> Sum/2
  Sqrt/1 -> Out1/1
  Math Function/1 -> Sum/1
  Unit Delay/1 -> Gain/1
  Gain1/1 -> Unit Delay/1, Sqrt/1
  Sum/1 -> Gain1/1
  In1/1 -> Math Function/1

== system afe_abc_inv_psm_2mods/afe_abc_inv_psm_mod2/AFE_control/afe_control/instantaneus_power/rms3 ==
  In1 : Inport
  Gain : Gain  Gain=n10-1
  Gain1 : Gain  Gain=1/n10
  Math Function : Math  Operator=magnitude^2  SignedPower=on
  Sqrt : Sqrt
  Sum : Sum  Inputs=|++
  Unit Delay : UnitDelay  SampleTime=-1  HasFrameUpgradeWarning=on
  Out1 : Outport  VectorParamsAs1DForOutWhenUnconnected=off
  wires:
  In1/1 -> Math Function/1
  Sum/1 -> Gain1/1
  Gain1/1 -> Sqrt/1, Unit Delay/1
  Unit Delay/1 -> Gain/1
  Math Function/1 -> Sum/1
  Sqrt/1 -> Out1/1
  Gain/1 -> Sum/2

== system afe_abc_inv_psm_2mods/afe_abc_inv_psm_mod2/AFE_control/afe_control/instantaneus_power/rms4 ==
  In1 : Inport
  Gain : Gain  Gain=n10-1
  Gain1 : Gain  Gain=1/n10
  Math Function : Math  Operator=magnitude^2  SignedPower=on
  Sqrt : Sqrt
  Sum : Sum  Inputs=|++
  Unit Delay : UnitDelay  SampleTime=-1  HasFrameUpgradeWarning=on
  Out1 : Outport  VectorParamsAs1DForOutWhenUnconnected=off
  wires:
  Gain/1 -> Sum/2
  Sqrt/1 -> Out1/1
  Math Function/1 -> Sum/1
  Unit Delay/1 -> Gain/1
  Gain1/1 -> Unit Delay/1, Sqrt/1
  Sum/1 -> Gain1/1
  In1/1 -> Math Function/1

== system afe_abc_inv_psm_2mods/afe_abc_inv_psm_mod2/AFE_control/afe_control/instantaneus_power/rms5 ==
  In1 : Inport
  Gain : Gain  Gain=n10-1
  Gain1 : Gain  Gain=1/n10
  Math Function : Math  Operator=magnitude^2  SignedPower=on
  Sqrt : Sqrt
  Sum : Sum  Inputs=|++
  Unit Delay : UnitDelay  SampleTime=-1  HasFrameUpgradeWarning=on
  Out1 : Outport  VectorParamsAs1DForOutWhenUnconnected=off
  wires:
  In1/1 -> Math Function/1
  Sum/1 -> Gain1/1
  Gain1/1 -> Sqrt/1, Unit Delay/1
  Unit Delay/1 -> Gain/1
  Math Function/1 -> Sum/1
  Sqrt/1 -> Out1/1
  Gain/1 -> Sum/2

== system afe_abc_inv_psm_2mods/afe_abc_inv_psm_mod2/AFE_control/afe_control/is afe quantizzation and one step delay/is afe quantizzation and one step delay ==
  is_u_pu : Inport
  is_v_pu : Inport  Port=2
  is_w_pu : Inport  Port=3
  Quantizer : Quantizer  QuantizationInterval=adc_quantization
  Quantizer1 : Quantizer  QuantizationInterval=adc_quantization
  Quantizer2 : Quantizer  QuantizationInterval=adc_quantization
  Unit Delay : UnitDelay  SampleTime=-1  HasFrameUpgradeWarning=on
  Unit Delay1 : UnitDelay  SampleTime=-1  HasFrameUpgradeWarning=on
  Unit Delay2 : UnitDelay  SampleTime=-1  HasFrameUpgradeWarning=on
  isd_u_pu : Outport
  isd_v_pu : Outport  Port=2
  isd_w_pu : Outport  Port=3
  wires:
  is_w_pu/1 -> Quantizer2/1
  is_v_pu/1 -> Quantizer1/1
  is_u_pu/1 -> Quantizer/1
  Quantizer2/1 -> Unit Delay2/1
  Quantizer1/1 -> Unit Delay1/1
  Quantizer/1 -> Unit Delay/1
  Unit Delay2/1 -> isd_w_pu/1
  Unit Delay1/1 -> isd_v_pu/1
  Unit Delay/1 -> isd_u_pu/1

== system afe_abc_inv_psm_2mods/afe_abc_inv_psm_mod2/AFE_control/afe_control/islanding_mode_detector/moving_avarage_1 ==
  u : Inport
  Abs : Abs  SaturateOnIntegerOverflow=off
  Constant : Constant
  Constant1 : Constant  Value=ts_afe
  Gain : Gain  Gain=w_grid
  MATLAB Function1 : MATLAB Function  TreatAsAtomicUnit=on
  Saturation : Saturate  UpperLimit=2  LowerLimit=0.1
  Unit Delay : UnitDelay  SampleTime=-1  HasFrameUpgradeWarning=on
  y : Outport
  wires:
  Gain/1 -> MATLAB Function1/3(omega)
  [omega_grid_pll_mod2] -> Abs/1
  Abs/1 -> Saturation/1
  Saturation/1 -> Gain/1
  Constant1/1 -> MATLAB Function1/5(ts)
  Constant/1 -> MATLAB Function1/4(nperiods)
  MATLAB Function1/1(y) -> Unit Delay/1
  Unit Delay/1 -> MATLAB Function1/1(y_1), y/1
  u/1 -> MATLAB Function1/2(u)

== system afe_abc_inv_psm_2mods/afe_abc_inv_psm_mod2/AFE_control/afe_control/islanding_mode_detector/moving_avarage_2 ==
  u : Inport
  Abs : Abs  SaturateOnIntegerOverflow=off
  Constant : Constant
  Constant1 : Constant  Value=ts_afe
  Gain : Gain  Gain=w_grid
  MATLAB Function1 : MATLAB Function  TreatAsAtomicUnit=on
  Saturation : Saturate  UpperLimit=2  LowerLimit=0.1
  Unit Delay : UnitDelay  SampleTime=-1  HasFrameUpgradeWarning=on
  y : Outport
  wires:
  Gain/1 -> MATLAB Function1/3(omega)
  [omega_grid_pll_mod2] -> Abs/1
  u/1 -> MATLAB Function1/2(u)
  Unit Delay/1 -> y/1, MATLAB Function1/1(y_1)
  MATLAB Function1/1(y) -> Unit Delay/1
  Constant/1 -> MATLAB Function1/4(nperiods)
  Constant1/1 -> MATLAB Function1/5(ts)
  Saturation/1 -> Gain/1
  Abs/1 -> Saturation/1

== system afe_abc_inv_psm_2mods/afe_abc_inv_psm_mod2/AFE_control/afe_control/phase_compensation_1/alignment_ctrl ==
  local_time : Inport
  master_time : Inport  Port=2
  Constant : Constant  Value=0
  Gain : Gain  Gain=-1
  Sum : Sum  Inputs=|+-
  pi : Subsystem  mask{kp=kp_align, ki=ki_align, lim_up=lim_up_align, lim_down=lim_down_align}
      mask prompts: ki "ki*ts"
      mask Display:
      | disp('pi()');
      | port_label('input', 1, 'u_ref');
      | port_label('input', 2, 'u');
      | port_label('output', 1, 'y');
  dp : Outport
  wires:
  master_time/1 -> Sum/1
  Sum/1 -> Gain/1
  Constant/1 -> pi/1(u_ref)
  local_time/1 -> Sum/2
  Gain/1 -> pi/2(u)
  pi/1(y) -> dp/1

== system afe_abc_inv_psm_2mods/afe_abc_inv_psm_mod2/AFE_control/afe_control/ug afe quantizzation and one step delay/ug afe quantizzation and one step delay ==
  ug_u_pu : Inport
  ug_v_pu : Inport  Port=2
  ug_w_pu : Inport  Port=3
  Quantizer1 : Quantizer  QuantizationInterval=adc_quantization
  Quantizer2 : Quantizer  QuantizationInterval=adc_quantization
  Quantizer4 : Quantizer  QuantizationInterval=adc_quantization
  Unit Delay : UnitDelay  SampleTime=-1  HasFrameUpgradeWarning=on
  Unit Delay1 : UnitDelay  SampleTime=-1  HasFrameUpgradeWarning=on
  Unit Delay2 : UnitDelay  SampleTime=-1  HasFrameUpgradeWarning=on
  ugd_u_pu : Outport
  ugd_v_pu : Outport  Port=2
  ugd_w_pu : Outport  Port=3
  wires:
  ug_u_pu/1 -> Quantizer4/1
  ug_v_pu/1 -> Quantizer1/1
  ug_w_pu/1 -> Quantizer2/1
  Quantizer2/1 -> Unit Delay2/1
  Quantizer1/1 -> Unit Delay1/1
  Quantizer4/1 -> Unit Delay/1
  Unit Delay2/1 -> ugd_w_pu/1
  Unit Delay1/1 -> ugd_v_pu/1
  Unit Delay/1 -> ugd_u_pu/1

== system afe_abc_inv_psm_2mods/afe_abc_inv_psm_mod2/INV_control/inverter_control/current_ctrl/bemf_observer ==
  ialpha_pu : Inport
  ibeta_pu : Inport  Port=2
  ualpha_pu : Inport  Port=3
  ubeta_pu : Inport  Port=4
  udc_pu : Inport  Port=5
  BEMF Observer simulink/Ccaller mod2 : Scope  NumInputPorts=2
      settings: ActiveDisplayYMinimum=-8.208439445506059  ActiveDisplayYMaximum=1.8110307694422199
  Mux : Mux  Inputs=3
  Mux1 : Mux  Inputs=3
  Variant Source : VariantSource  VariantControls={use_observer_from_simulink_module_2 == 1, use_observer_from_ccaller_module_2 == 1}
  Variant Source1 : VariantSource  VariantControls={use_observer_from_simulink_module_2 == 1, use_observer_from_ccaller_module_2 == 1}
  bemf_observer : Subsystem
  bemf_observer_ccaller : Subsystem  Commented=on
  phase_fault : Subsystem  Commented=on
  tag scope: omega_hat_pu_mod2=global, theta_hat_mod2=global
  wires:
  udc_pu/1 -> bemf_observer/5(udc_pu), bemf_observer_ccaller/5(udc_pu)
  phase_fault/2(theta_hat_encoder) -> Mux1/3
  phase_fault/1(omega_pu_encoder) -> Mux/3
  Variant Source/1 -> [omega_hat_pu_mod2]
  Variant Source1/1 -> [theta_hat_mod2]
  bemf_observer/2(theta_hat) -> Mux1/1, Variant Source1/1  "theta_hat"
  bemf_observer_ccaller/1(omega_pu) -> Variant Source/2, Mux/2  "omega_pu_code"
  bemf_observer_ccaller/2(theta_hat) -> Variant Source1/2, Mux1/2  "theta_hat_code"
  bemf_observer/1(omega_pu) -> Mux/1, Variant Source/1  "omega_pu"
  ubeta_pu/1 -> bemf_observer/4(ubeta_pu), bemf_observer_ccaller/4(ubeta_pu)
  ualpha_pu/1 -> bemf_observer/3(ualpha_pu), bemf_observer_ccaller/3(ualpha_pu)
  Mux1/1 -> BEMF Observer simulink/Ccaller mod2/2
  Mux/1 -> BEMF Observer simulink/Ccaller mod2/1
  ibeta_pu/1 -> bemf_observer/2(ibeta_pu), bemf_observer_ccaller/2(ibeta_pu)
  ialpha_pu/1 -> bemf_observer_ccaller/1(ialpha_pu), bemf_observer/1(ialpha_pu)

== system afe_abc_inv_psm_2mods/afe_abc_inv_psm_mod2/INV_control/inverter_control/current_ctrl/current_ctrl ==
  iq_ref : Inport
  udc_pu : Inport  Port=2
  MTPA _mod1 : Subsystem
  Sqrt : Sqrt
  Square : Math  Operator=square
  Square1 : Math  Operator=square
  Sum : Sum  Inputs=|++
  Unit Delay2 : UnitDelay  SampleTime=-1  HasFrameUpgradeWarning=on
  Unit Delay3 : UnitDelay  SampleTime=-1  HasFrameUpgradeWarning=on
  dq2alphabeta : MATLAB Function  TreatAsAtomicUnit=on
  dq_pi_with_vector_antiwindup mod2 : Subsystem
  id_ref _mod1 : Subsystem
      settings: PortSchema="{\"entries\":[{\"content\":{\"sides\":[{\"content\":{},\"type\":\"ConnectorPlacement.EquallySpacedRectSide\",\"uuid\":\"42af5d69-f0eb-42c6-9e03-28c1d0757323\"},{\"content\":{\"connectorIds\":[\"Out1\"],\"side\":\"RIGHT\"},\"type\":\"ConnectorPlacement.EquallySpacedRectSide\",\"uuid\":\"dd68a9f9-d15f-4e57-9d9e-130889a7b90c\"},{\"content\":{\"connectorIds\":[\"In1\"],\"side\":\"TOP\"},\"type\":\"ConnectorPlacement.EquallySpacedRectSide\",\"uuid\":\"68c797a2-8439-4b8d-8368-b7485adf0676\"}]},\"type\":\"ConnectorPlacement.EquallySpacedConnector\",\"uuid\":\"693c5f1c-0580-4626-8f13-b27865dfb3ac\"}],\"packageUris\":[\"http://schema.mathworks.com/mf0/Connector/R2020b\"],\"version\":\"1.0\"}"
  idref/id mod2 : Scope  NumInputPorts=2
      settings: ActiveDisplayYMinimum=-0.6792366431007606  ActiveDisplayYMaximum=0.075577635851628425
  iqref/iq mod2 : Scope  NumInputPorts=2
      settings: ActiveDisplayYMinimum=-0.97391738160095387  ActiveDisplayYMaximum=0.10821304240010596  DataLoggingVariableName=ScopeData2
  tag scope: id_pu_ref_mod2=global, iq_pu_ref_mod2=global, u_mot_pu_mod2=global, ualpha_pu_mod2=global, ubeta_pu_mod2=global, ud_pu_mod2=global, uq_pu_mod2=global
  wires:
  dq2alphabeta/2(beta) -> Unit Delay3/1
  [theta_hat_mod2] -> dq2alphabeta/3(gamma)
  Unit Delay3/1 -> [ubeta_pu_mod2]
  Unit Delay2/1 -> [ualpha_pu_mod2]
  dq2alphabeta/1(alpha) -> Unit Delay2/1
  [ud_pu_mod2] -> dq2alphabeta/1(d)
  [uq_pu_mod2] -> dq2alphabeta/2(q)
  udc_pu/1 -> dq_pi_with_vector_antiwindup mod2/5(udc_pu)
  id_ref _mod1/1(id_ref) -> dq_pi_with_vector_antiwindup mod2/1(id_ref), idref/id mod2/1
  Sqrt/1 -> [u_mot_pu_mod2]
  Square1/1 -> Sum/2
  Sum/1 -> Sqrt/1
  Square/1 -> Sum/1
  dq_pi_with_vector_antiwindup mod2/2(ctrl_q_u) -> Square/1, [uq_pu_mod2]
  dq_pi_with_vector_antiwindup mod2/1(ctrl_d_u) -> Square1/1, [ud_pu_mod2]
  iq_ref/1 -> [iq_pu_ref_mod2], dq_pi_with_vector_antiwindup mod2/3(iq_ref), iqref/iq mod2/1, MTPA _mod1/1(iq_ref)  "iq_ref"
  MTPA _mod1/1(Id_ref_mtpa) -> [id_pu_ref_mod2], id_ref _mod1/1(id_mtpa)  "id_ref"
  [id_pu_mod2] -> dq_pi_with_vector_antiwindup mod2/2(id), idref/id mod2/2  "id"
  [iq_pu_mod2] -> dq_pi_with_vector_antiwindup mod2/4(iq), iqref/iq mod2/2  "iq"

== system afe_abc_inv_psm_2mods/afe_abc_inv_psm_mod2/INV_control/inverter_control/current_ctrl/current_transformation ==
  Demux : Demux  Outputs=3
  alphabeta2dq : MATLAB Function  TreatAsAtomicUnit=on
  uvw2alphabeta : MATLAB Function  TreatAsAtomicUnit=on
  tag scope: ialpha_pu_mod2=global, ibeta_pu_mod2=global, id_pu_mod2=global, iq_pu_mod2=global
  wires:
  [isd_uvw_inv_mod2] -> Demux/1
  Demux/1 -> uvw2alphabeta/1(u)  "iu"
  Demux/2 -> uvw2alphabeta/2(v)  "iv"
  Demux/3 -> uvw2alphabeta/3(w)  "iw"
  [theta_hat_mod2] -> alphabeta2dq/3(gamma)
  uvw2alphabeta/1(alpha) -> alphabeta2dq/1(alpha), [ialpha_pu_mod2]  "ialpha_pu"
  uvw2alphabeta/2(beta) -> alphabeta2dq/2(beta), [ibeta_pu_mod2]  "ibeta_pu"
  alphabeta2dq/1(d) -> [id_pu_mod2]  "id_pu"
  alphabeta2dq/2(q) -> [iq_pu_mod2]  "iq_pu"
